simulink model "Nonlinear_System_Swingup"  (R2020a)
settings: Solver=ode4  StartTime=0.0  StopTime=10  FixedStep=.0001  RelTol=1e-3
values from neighbouring files (symbols this model uses):
  g = 9.81    [parameters.m]
  I_bar_1_z1 = 0.00086    [parameters.m]
  I_bar_2_x2 = 9.0257e-4    (= 0.00090257)    [parameters.m]
  I_bar_2_x2y2 = 2.265e-5    (= 2.265e-05)    [parameters.m]
  I_bar_2_y2 = 9.31e-6    (= 9.31e-06)    [parameters.m]
  I_bar_2_z2 = 9.102e-4    (= 0.0009102)    [parameters.m]
  Kt = 0.0833    [parameters.m]
  L1 = 0.2032    [parameters.m]
  L11 = 0.0051    [parameters.m]
  L21 = 0.083    [parameters.m]
  M1 = 0.312    [parameters.m]
  M2 = 0.0787    [parameters.m]
libraries: simulink x2
settings Model: EnablePacing=on  Creator=Aditya  LastModifiedBy=nikhita
settings SolverCC: AlgebraicLoopSolver=LineSearch
settings DebuggingCC: AlgebraicLoopMsg=none  ArithmeticOperatorsInVariantConditions=warning
settings SFSimCC: CustomCodeUndefinedFunction=UseInterfaceOnly

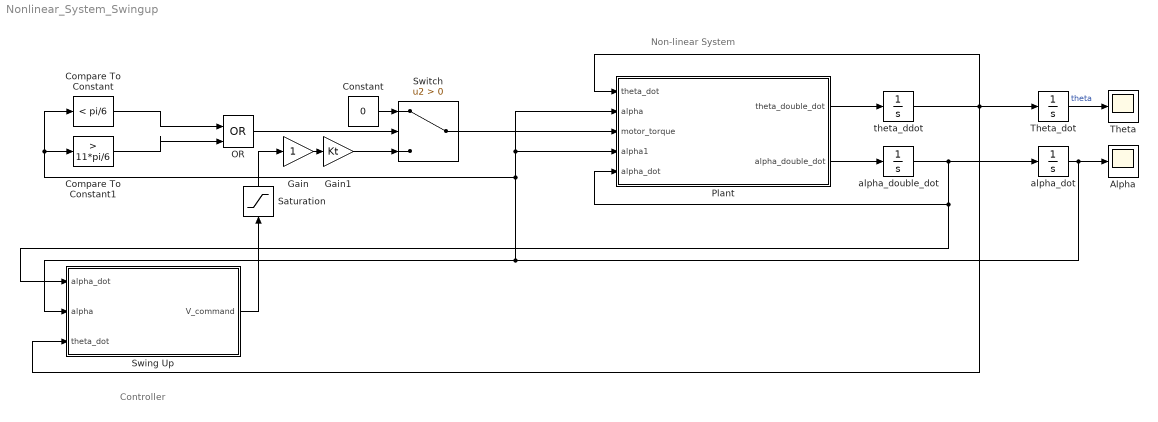
== system Nonlinear_System_Swingup ==
  note: Non-linear System
  note: Controller
  Alpha : Scope
  Compare To Constant : simulink/Logic and Bit Operations/Compare To Constant  relop=<  const=pi/6  OutDataTypeStr=boolean
  Compare To Constant1 : simulink/Logic and Bit Operations/Compare To Constant  relop=>  const=11*pi/6  OutDataTypeStr=boolean
  Constant : Constant  Value=0
  Gain : Gain
  Gain1 : Gain  Gain=Kt
  OR : Logic  Operator=OR  IconShape=distinctive  AllPortsSameDT=off  OutDataTypeStr=boolean
  Plant : Subsystem
  Saturation : Saturate  UpperLimit=3  LowerLimit=-3
  "Swing Up " : Subsystem
  Switch : Switch  Criteria=u2 > Threshold
  Theta : Scope
  Theta_dot : Integrator
  alpha_dot : Integrator  InitialCondition=pi+.1
  alpha_double_dot : Integrator
  theta_ddot : Integrator
  wires:
  theta_ddot/1 -> "Swing Up "/3(theta_dot), Theta_dot/1, Plant/1(theta_dot)
  Theta_dot/1 -> Theta/1  "theta"
  alpha_double_dot/1 -> "Swing Up "/1(alpha_dot), Plant/5(alpha_dot), alpha_dot/1
  "Swing Up "/1(V_command) -> Saturation/1
  Gain/1 -> Gain1/1
  alpha_dot/1 -> Alpha/1, "Swing Up "/2(alpha), Plant/2(alpha), Plant/4(alpha1), Compare To Constant/1, Compare To Constant1/1
  OR/1 -> Switch/2
  Compare To Constant1/1 -> OR/2
  Compare To Constant/1 -> OR/1
  Gain1/1 -> Switch/3
  Constant/1 -> Switch/1
  Saturation/1 -> Gain/1
  Switch/1 -> Plant/3("motor_torque ")
  Plant/1("theta_double_dot ") -> theta_ddot/1
  Plant/2(alpha_double_dot) -> alpha_double_dot/1

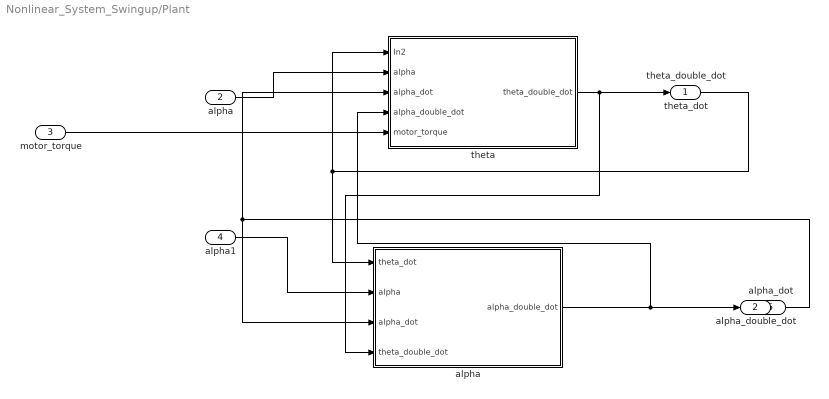
== system Nonlinear_System_Swingup/Plant ==
  theta_dot : Inport
  alpha : Inport  Port=2
  "motor_torque " : Inport  Port=3
  alpha1 : Inport  Port=4
  alpha_dot : Inport  Port=5
  "alpha " : Subsystem
  "theta " : Subsystem
  "theta_double_dot " : Outport
  alpha_double_dot : Outport  Port=2
  wires:
  "motor_torque "/1 -> "theta "/5("motor_torque ")
  theta_dot/1 -> "alpha "/1(theta_dot), "theta "/1(In2)
  alpha/1 -> "theta "/2(alpha)
  alpha1/1 -> "alpha "/2(alpha)
  "alpha "/1(alpha_double_dot) -> alpha_double_dot/1, "theta "/4(alpha_double_dot)
  alpha_dot/1 -> "theta "/3(alpha_dot), "alpha "/3(alpha_dot)
  "theta "/1("theta_double_dot ") -> "theta_double_dot "/1, "alpha "/4(theta_double_dot)

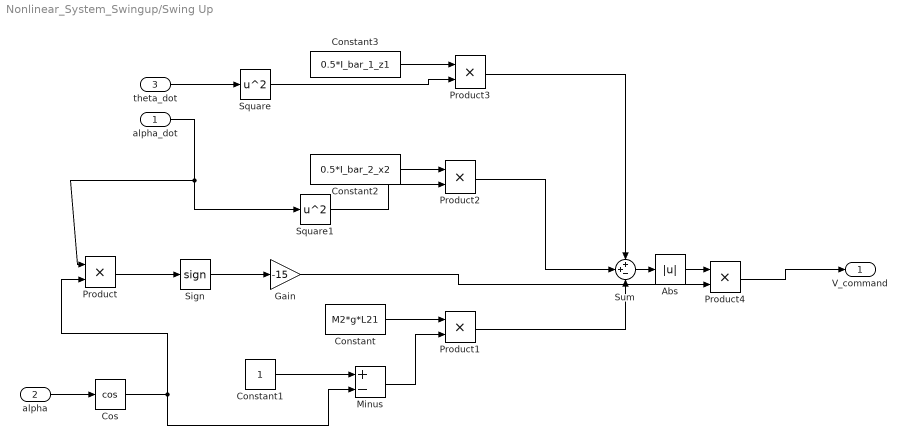
== system Nonlinear_System_Swingup/Swing Up  ==
  alpha_dot : Inport
  alpha : Inport  Port=2
  theta_dot : Inport  Port=3
  Abs : Abs
  Constant : Constant  Value=M2*g*L21
  Constant1 : Constant
  Constant2 : Constant  Value=0.5*I_bar_2_x2
  Constant3 : Constant  Value=0.5*I_bar_1_z1
  Cos : Trigonometry  Operator=cos
  Gain : Gain  Gain=-15
  Minus : Sum  Inputs=+-
  Product{,1..4} (5 alike) : Product
  Sign : Signum
  Square : Math  Operator=square  SignedPower=on  SaturateOnIntegerOverflow=on
  Square1 : Math  Operator=square  SignedPower=on  SaturateOnIntegerOverflow=on
  Sum : Sum  Inputs=++-
  V_command : Outport  VectorParamsAs1DForOutWhenUnconnected=off
  wires:
  alpha_dot/1 -> Square1/1, Product/1
  alpha/1 -> Cos/1
  Product/1 -> Sign/1
  Cos/1 -> Minus/2, Product/2
  Sign/1 -> Gain/1
  Constant/1 -> Product1/1
  Constant1/1 -> Minus/1
  Minus/1 -> Product1/2
  Product1/1 -> Sum/3
  Constant2/1 -> Product2/1
  Constant3/1 -> Product3/1
  theta_dot/1 -> Square/1
  Product3/1 -> Sum/1
  Product2/1 -> Sum/2
  Square/1 -> Product3/2
  Square1/1 -> Product2/2
  Sum/1 -> Abs/1
  Gain/1 -> Product4/2
  Product4/1 -> V_command/1
  Abs/1 -> Product4/1

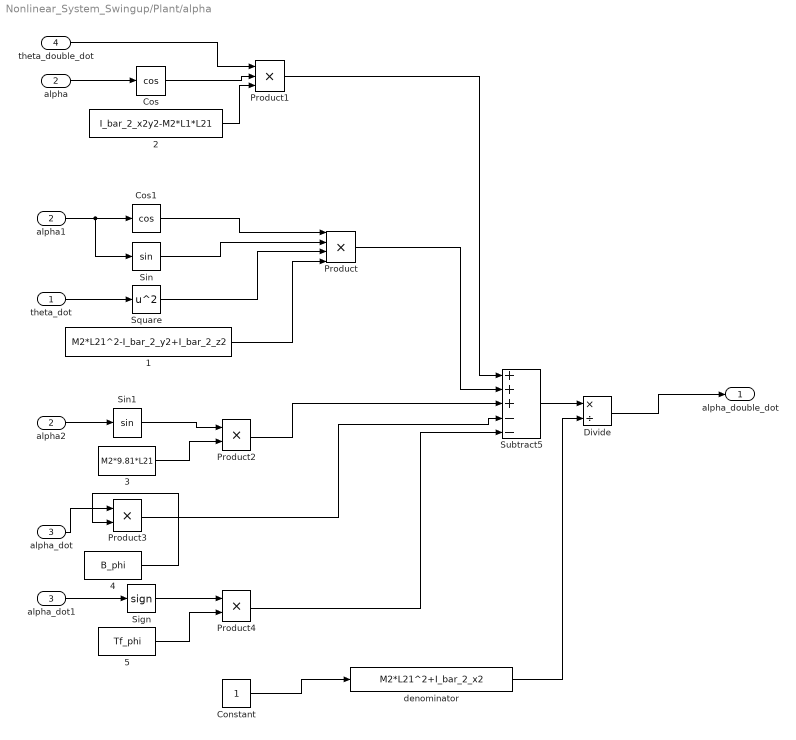
== system Nonlinear_System_Swingup/Plant/alpha  ==
  theta_dot : Inport
  alpha : Inport  Port=2
  alpha_dot : Inport  Port=3
  theta_double_dot : Inport  Port=4
  1 : Fcn  Expr=M2*L21^2-I_bar_2_y2+I_bar_2_z2
  2 : Fcn  Expr=I_bar_2_x2y2-M2*L1*L21
  3 : Fcn  Expr=M2*9.81*L21
  4 : Fcn  Expr=B_phi
  5 : Fcn  Expr=Tf_phi
  Constant : Constant
  Cos : Trigonometry  Operator=cos
  Cos1 : Trigonometry  Operator=cos
  Divide : Product  Inputs=*/
  Product : Product  Inputs=4
  Product1 : Product  Inputs=3
  Product2 : Product
  Product3 : Product
  Product4 : Product
  Sign : Signum
  Sin : Trigonometry
  Sin1 : Trigonometry
  Square : Math  Operator=square  SignedPower=on  SaturateOnIntegerOverflow=on
  Subtract5 : Sum  Inputs=+++--
  alpha1 : InportShadow  Port=2
  alpha2 : InportShadow  Port=2
  alpha_dot1 : InportShadow  Port=3
  "denominator " : Fcn  Expr=M2*L21^2+I_bar_2_x2
  alpha_double_dot : Outport
  wires:
  alpha/1 -> Cos/1
  alpha1/1 -> Sin/1, Cos1/1
  theta_dot/1 -> Square/1
  Sin/1 -> Product/2
  Cos1/1 -> Product/1
  Cos/1 -> Product1/2
  theta_double_dot/1 -> Product1/1
  Square/1 -> Product/3
  alpha2/1 -> Sin1/1
  Sin1/1 -> Product2/1
  alpha_dot/1 -> Product3/1
  alpha_dot1/1 -> Sign/1
  Product1/1 -> Subtract5/1
  Product/1 -> Subtract5/2
  Product2/1 -> Subtract5/3
  Product3/1 -> Subtract5/4
  Product4/1 -> Subtract5/5
  Subtract5/1 -> Divide/1
  "denominator "/1 -> Divide/2
  Divide/1 -> alpha_double_dot/1
  Sign/1 -> Product4/1
  Constant/1 -> "denominator "/1
  3/1 -> Product2/2
  1/1 -> Product/4
  2/1 -> Product1/3
  4/1 -> Product3/2
  5/1 -> Product4/2

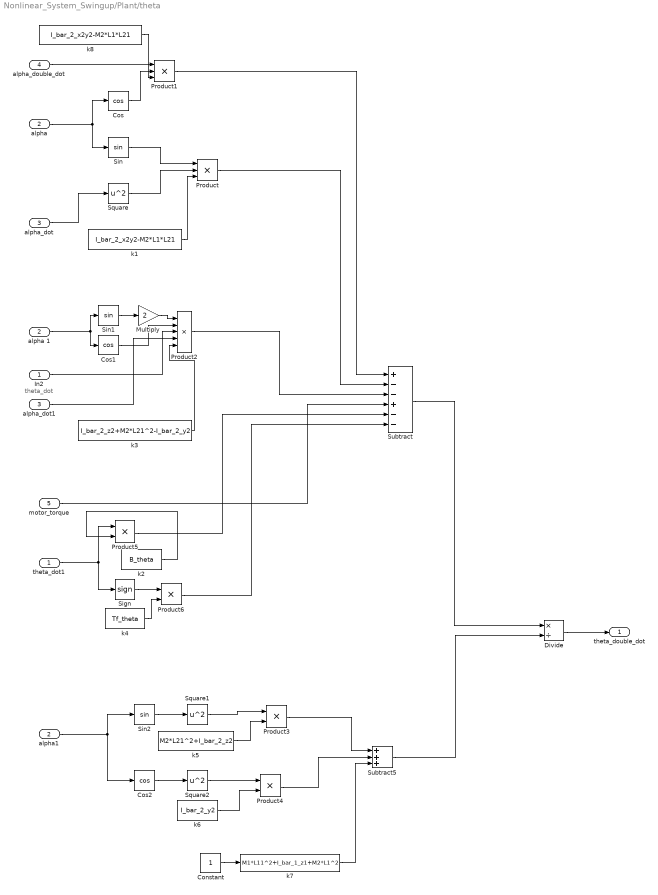
== system Nonlinear_System_Swingup/Plant/theta  ==
  note: theta_dot
  In2 : Inport
  alpha : Inport  Port=2
  alpha_dot : Inport  Port=3
  alpha_double_dot : Inport  Port=4
  "motor_torque " : Inport  Port=5
  Constant : Constant
  Cos : Trigonometry  Operator=cos
  Cos1 : Trigonometry  Operator=cos
  Cos2 : Trigonometry  Operator=cos
  Divide : Product  Inputs=*/
  Multiply : Gain  Gain=2
  Product : Product  Inputs=3
  Product1 : Product  Inputs=3
  Product2 : Product  Inputs=5
  Product{3..6} (4 alike) : Product
  Sign : Signum
  Sin : Trigonometry
  Sin1 : Trigonometry
  Sin2 : Trigonometry
  Square : Math  Operator=square  SignedPower=on  SaturateOnIntegerOverflow=on
  Square1 : Math  Operator=square  SignedPower=on  SaturateOnIntegerOverflow=on
  Square2 : Math  Operator=square  SignedPower=on  SaturateOnIntegerOverflow=on
  Subtract : Sum  Inputs=+--+--
  Subtract5 : Sum  Inputs=+++
  alpha 1 : InportShadow  Port=2
  alpha1 : InportShadow  Port=2
  alpha_dot1 : InportShadow  Port=3
  k1 : Fcn  Expr=I_bar_2_x2y2-M2*L1*L21
  k2 : Fcn  Expr=B_theta
  k3 : Fcn  Expr=I_bar_2_z2+M2*L21^2-I_bar_2_y2
  k4 : Fcn  Expr=Tf_theta
  k5 : Fcn  Expr=M2*L21^2+I_bar_2_z2
  k6 : Fcn  Expr=I_bar_2_y2
  k7 : Fcn  Expr=M1*L11^2+I_bar_1_z1+M2*L1^2
  k8 : Fcn  Expr=I_bar_2_x2y2-M2*L1*L21
  theta_dot1 : InportShadow
  "theta_double_dot " : Outport
  wires:
  alpha/1 -> Sin/1, Cos/1
  alpha_double_dot/1 -> Product1/1
  Cos/1 -> Product1/2
  alpha_dot/1 -> Square/1
  Sin/1 -> Product/1
  Square/1 -> Product/2
  Cos1/1 -> Product2/2
  Sin1/1 -> Multiply/1
  In2/1 -> Product2/3
  alpha_dot1/1 -> Product2/4
  theta_dot1/1 -> Product5/1, Sign/1
  Sign/1 -> Product6/1
  "motor_torque "/1 -> Subtract/4
  Product5/1 -> Subtract/5
  Product6/1 -> Subtract/6
  Cos2/1 -> Square2/1
  Sin2/1 -> Square1/1
  alpha1/1 -> Cos2/1, Sin2/1
  Square1/1 -> Product3/1
  Square2/1 -> Product4/1
  k7/1 -> Subtract5/3
  Subtract/1 -> Divide/1
  Subtract5/1 -> Divide/2
  Divide/1 -> "theta_double_dot "/1
  Constant/1 -> k7/1
  Product/1 -> Subtract/2
  Product1/1 -> Subtract/1
  alpha 1/1 -> Cos1/1, Sin1/1
  Product2/1 -> Subtract/3
  Product3/1 -> Subtract5/1
  Product4/1 -> Subtract5/2
  Multiply/1 -> Product2/1
  k1/1 -> Product/3
  k8/1 -> Product1/3
  k3/1 -> Product2/5
  k6/1 -> Product4/2
  k5/1 -> Product3/2
  k4/1 -> Product6/2
  k2/1 -> Product5/2
